simulink model "RLSim5"  (R2015b)
settings: Solver=ode45  StartTime=0.0  StopTime=16435  MaxStep=1  RelTol=1e-3
libraries: simulink x1
settings Model: Creator=jeff  LastModifiedBy=jeff
settings SolverCC: ZeroCrossAlgorithm=Adaptive
settings DataIOCC: SaveFormat=Array
settings DebuggingCC: IgnoredZcDiagnostic=none  SolverPrmCheckMsg=warning
settings HardwareCC: ProdBitPerPointer=32  ProdLargestAtomicFloat=None  ProdIntDivRoundTo=Undefined  ProdEndianess=Unspecified  ProdWordSize=32  ProdHWDeviceType=32-bit Generic
settings GRTTargetCC: GeneratePreprocessorConditionals=Disable all
settings ConfigComp: CovModelRefEnable=Off  CovSFcnEnable=off

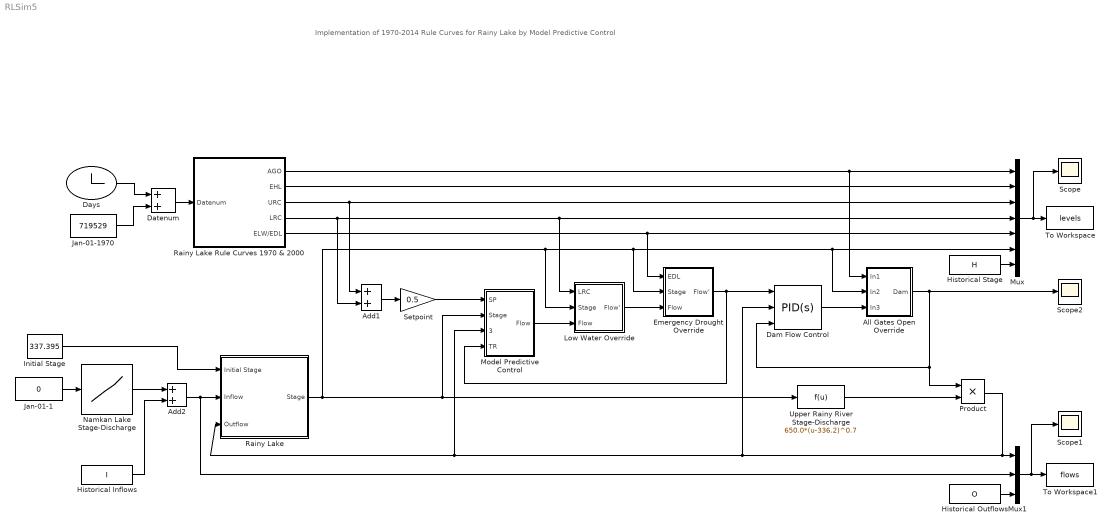
== system RLSim5 ==
  note: Implementation of 1970-2014 Rule Curves
      | for Rainy Lake by Model Predictive Control
  Add1 : Sum
  Add2 : Sum
  All Gates Open Override : Subsystem
  Dam Flow Control : simulink/Continuous/PID Controller (2DOF)  Controller=PID  TimeDomain=Continuous-time  SampleTime=-1  IntegratorMethod=Forward Euler  FilterMethod=Forward Euler  Form=Parallel  UseFilter=on  ControllerParametersSource=internal  P=0  I=0.00566146868750982  D=0  N=100  b=1  c=1  InitialConditionSource=internal  InitialConditionForIntegrator=0  InitialConditionForFilter=0  ExternalReset=none  LimitOutput=on  UpperSaturationLimit=1  LowerSaturationLimit=0  LinearizeAsGain=off  AntiWindupMode=clamping  Kb=1  TrackingMode=on  Kt=1  PParamMin=[]  PParamMax=[]  IParamMin=[]  IParamMax=[]  DParamMin=[]  DParamMax=[]  NParamMin=[]  NParamMax=[]  bParamMin=[]  bParamMax=[]  cParamMin=[]  cParamMax=[]  KbParamMin=[]  KbParamMax=[]  KtParamMin=[]  KtParamMax=[]  POutMin=[]  POutMax=[]  IOutMin=[]  IOutMax=[]  DOutMin=[]  DOutMax=[]  NOutMin=[]  NOutMax=[]  bOutMin=[]  bOutMax=[]  cOutMin=[]  cOutMax=[]  KbOutMin=[]  KbOutMax=[]  KtOutMin=[]  KtOutMax=[]  IntegratorOutMin=[]  IntegratorOutMax=[]  FilterOutMin=[]  FilterOutMax=[]  SumOutMin=[]  SumOutMax=[]  Sum1OutMin=[]  Sum1OutMax=[]  Sum2OutMin=[]  Sum2OutMax=[]  Sum3OutMin=[]  Sum3OutMax=[]  SumI1OutMin=[]  SumI1OutMax=[]  SumI2OutMin=[]  SumI2OutMax=[]  SumI3OutMin=[]  SumI3OutMax=[]  SumDOutMin=[]  SumDOutMax=[]  SaturationOutMin=[]  SaturationOutMax=[]  IntegratorContinuousStateAttributes=''  IntegratorStateMustResolveToSignalObject=off  IntegratorRTWStateStorageClass=Auto  FilterContinuousStateAttributes=''  FilterStateMustResolveToSignalObject=off  FilterRTWStateStorageClass=Auto  DifferentiatorICPrevScaledInput=0  DifferentiatorOutMin=[]  DifferentiatorOutMax=[]
  Datenum : Sum
  Days : Clock
  Emergency Drought Override : Subsystem
  Historical Inflows : FromWorkspace  VariableName=I  SampleTime=1
  Historical Outflows : FromWorkspace  VariableName=O  SampleTime=1
  Historical Stage : FromWorkspace  VariableName=H  SampleTime=1
  Initial Stage : Constant  Value=337.395
  Jan-01-1 : Constant  Value=0
  Jan-01-1970 : Constant  Value=719529
  Low Water Override : Subsystem
  Model Predictive Control : Subsystem
  Mux : Mux  Inputs=7
  Mux1 : Mux  Inputs=3
  Namkan Lake Stage-Discharge : Lookup_n-D  NumberOfTableDimensions=1  BreakpointsForDimension1=[335.21, 337.0, 338.0, 338.5, 339.0, 339.5, 340.0, 340.5, 341.0, 341.5, 342.0, 342.5, 343.0]  Table=[0 51 120 173 233 299 373 455 549 659 772 886 999]  ExtrapMethod=Clip  InternalRulePriority=Speed  RndMeth=Simplest  InputSameDT=on
  Product : Product
  Rainy Lake : Subsystem
  Rainy Lake Rule Curves 1970 & 2000 : Subsystem
  Scope : Scope
  Scope1 : Scope
  Scope2 : Scope
  Setpoint : Gain  Gain=0.5
  To Workspace : ToWorkspace  VariableName=levels  SaveFormat=Timeseries  SampleTime=-1
  To Workspace1 : ToWorkspace  VariableName=flows  SaveFormat=Timeseries  SampleTime=-1
  Upper Rainy River Stage-Discharge : Fcn  Expr=650.0*(u-336.2)^0.7
  wires:
  Days/1 -> Datenum/1
  Jan-01-1970/1 -> Datenum/2
  Datenum/1 -> Rainy Lake Rule Curves 1970 & 2000/1(Datenum)
  Mux/1 -> Scope/1, To Workspace/1
  Add1/1 -> Setpoint/1
  Rainy Lake Rule Curves 1970 & 2000/3(URC) -> Mux/3, Add1/1
  Initial Stage/1 -> Rainy Lake/1(Initial Stage)
  Mux1/1 -> Scope1/1, To Workspace1/1
  Rainy Lake Rule Curves 1970 & 2000/1(AGO) -> All Gates Open Override/1(In1), Mux/1
  Historical Stage/1 -> Mux/7
  Historical Outflows/1 -> Mux1/3
  Rainy Lake Rule Curves 1970 & 2000/2(EHL) -> Mux/2
  Add2/1 -> Mux1/2, Rainy Lake/2(Inflow)
  Namkan Lake Stage-Discharge/1 -> Add2/1
  Historical Inflows/1 -> Add2/2
  Jan-01-1/1 -> Namkan Lake Stage-Discharge/1
  Upper Rainy River Stage-Discharge/1 -> Product/2
  Product/1 -> Rainy Lake/3(Outflow), Model Predictive Control/3(Outflow), Dam Flow Control/2, Mux1/1
  Rainy Lake Rule Curves 1970 & 2000/5(ELW/EDL) -> Mux/5, Emergency Drought Override/1(EDL)
  Rainy Lake/1(Stage) -> Upper Rainy River Stage-Discharge/1, Model Predictive Control/2(Stage), Mux/6, All Gates Open Override/2(In2), Emergency Drought Override/2(Stage), Low Water Override/2(Stage)
  Low Water Override/1(Flow') -> Emergency Drought Override/3(Flow)
  Dam Flow Control/1 -> All Gates Open Override/3(In3)
  Emergency Drought Override/1(Flow') -> Dam Flow Control/1, Model Predictive Control/4(TR)
  Setpoint/1 -> Model Predictive Control/1(SP)
  Model Predictive Control/1(Flow) -> Low Water Override/3(Flow)
  Rainy Lake Rule Curves 1970 & 2000/4(LRC) -> Add1/2, Mux/4, Low Water Override/1(LRC)
  All Gates Open Override/1(Dam) -> Product/1, Dam Flow Control/3, Scope2/1

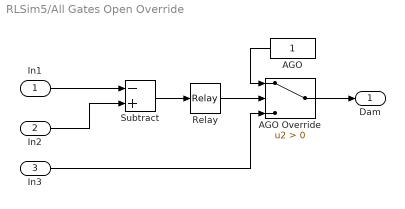
== system RLSim5/All Gates Open Override ==
  In1 : Inport
  In2 : Inport  Port=2
  In3 : Inport  Port=3
  AGO : Constant
  AGO Override : Switch  Criteria=u2 > Threshold
  Relay : Relay  OnSwitchValue=0.02  OffSwitchValue=-0.02
  Subtract : Sum  Inputs=-+
  Dam : Outport
  wires:
  Relay/1 -> AGO Override/2
  In3/1 -> AGO Override/3
  Subtract/1 -> Relay/1
  In2/1 -> Subtract/2
  AGO/1 -> AGO Override/1
  AGO Override/1 -> Dam/1
  In1/1 -> Subtract/1

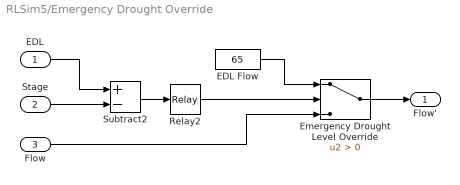
== system RLSim5/Emergency Drought Override ==
  EDL : Inport
  Stage : Inport  Port=2
  Flow : Inport  Port=3
  EDL Flow : Constant  Value=65
  Emergency Drought Level Override : Switch  Criteria=u2 > Threshold
  Relay2 : Relay  OnSwitchValue=0.02  OffSwitchValue=-0.02
  Subtract2 : Sum  Inputs=+-
  Flow' : Outport
  wires:
  Subtract2/1 -> Relay2/1
  Stage/1 -> Subtract2/2
  Emergency Drought Level Override/1 -> Flow'/1
  EDL Flow/1 -> Emergency Drought Level Override/1
  EDL/1 -> Subtract2/1
  Relay2/1 -> Emergency Drought Level Override/2
  Flow/1 -> Emergency Drought Level Override/3

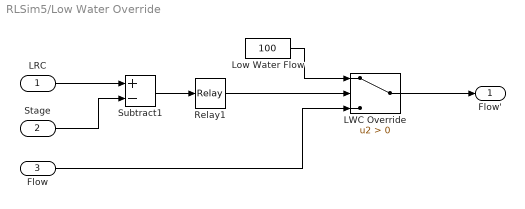
== system RLSim5/Low Water Override ==
  LRC : Inport
  Stage : Inport  Port=2
  Flow : Inport  Port=3
  LWC Override : Switch  Criteria=u2 > Threshold
  Low Water Flow : Constant  Value=100
  Relay1 : Relay  OnSwitchValue=0.02  OffSwitchValue=-0.02
  Subtract1 : Sum  Inputs=+-
  Flow' : Outport
  wires:
  Relay1/1 -> LWC Override/2
  Low Water Flow/1 -> LWC Override/1
  LWC Override/1 -> Flow'/1
  Subtract1/1 -> Relay1/1
  Flow/1 -> LWC Override/3
  LRC/1 -> Subtract1/1
  Stage/1 -> Subtract1/2

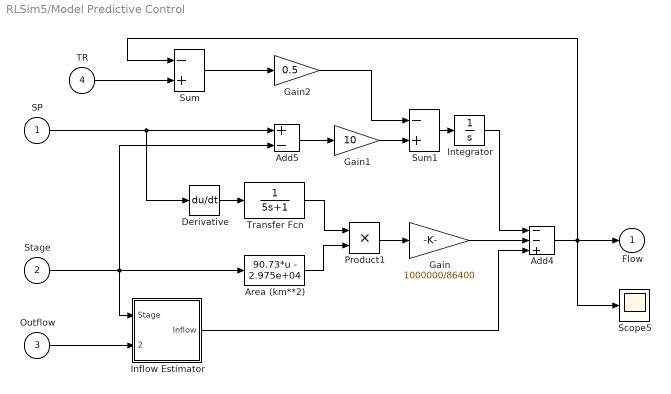
== system RLSim5/Model Predictive Control ==
  SP : Inport
  Stage : Inport  Port=2
  Outflow : Inport  Port=3
  TR : Inport  Port=4
  Add4 : Sum  Inputs=--+
  Add5 : Sum  Inputs=+-
  Area (km**2) : Fcn  Expr=90.73*u - 2.975e+04
  Derivative : Derivative  CoefficientInTFapproximation=Inf
  Gain : Gain  Gain=1000000/86400
  Gain1 : Gain  Gain=10
  Gain2 : Gain  Gain=0.5
  Inflow Estimator : Subsystem
  Integrator : Integrator
  Product1 : Product
  Scope5 : Scope
  Sum : Sum  Inputs=-+
  Sum1 : Sum  Inputs=-+
  Transfer Fcn : TransferFcn  Denominator=[5 1]
  Flow : Outport
  wires:
  Area (km**2)/1 -> Product1/2
  Stage/1 -> Add5/2, Area (km**2)/1, Inflow Estimator/1(Stage)
  SP/1 -> Derivative/1, Add5/1
  Add4/1 -> Flow/1, Scope5/1, Sum/1
  Add5/1 -> Gain1/1
  Product1/1 -> Gain/1
  Outflow/1 -> Inflow Estimator/2(Outflow)
  Derivative/1 -> Transfer Fcn/1
  Transfer Fcn/1 -> Product1/1
  Inflow Estimator/1(Inflow) -> Add4/3
  Gain/1 -> Add4/2
  Integrator/1 -> Add4/1
  TR/1 -> Sum/2
  Sum1/1 -> Integrator/1
  Gain1/1 -> Sum1/2
  Sum/1 -> Gain2/1
  Gain2/1 -> Sum1/1

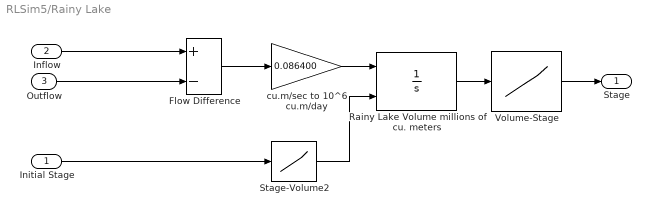
== system RLSim5/Rainy Lake ==
  Initial Stage : Inport
  Inflow : Inport  Port=2
  Outflow : Inport  Port=3
  Flow Difference : Sum  Inputs=+-
  Rainy Lake Volume millions of cu. meters : Integrator  InitialConditionSource=external  InitialCondition=1000  LimitOutput=on  LowerSaturationLimit=0  ContinuousStateAttributes='RainyLakeVolume'
  Stage-Volume2 : Lookup_n-D  NumberOfTableDimensions=1  BreakpointsForDimension1=[335.0 336.0 336.5 337.0 337.5 338.0 339.0 340.0]  Table=[112.67 798.00 1176.42 1577.25 2002.06 2450.57 3416.85 4458.97]  InternalRulePriority=Speed  RndMeth=Simplest  InputSameDT=on
  Volume-Stage : Lookup_n-D  NumberOfTableDimensions=1  BreakpointsForDimension1=[112.67 798.00 1176.42 1577.25 2002.06 2450.57 3416.85 4458.97]  Table=[335.0 336.0 336.5 337.0 337.5 338.0 339.0 340.0]  InternalRulePriority=Speed  RndMeth=Simplest  InputSameDT=on
  cu.m/sec to 10^6 cu.m/day : Gain  Gain=0.086400
  Stage : Outport
  wires:
  Outflow/1 -> Flow Difference/2
  Inflow/1 -> Flow Difference/1
  Rainy Lake Volume millions of cu. meters/1 -> Volume-Stage/1
  Stage-Volume2/1 -> Rainy Lake Volume millions of cu. meters/2
  cu.m/sec to 10^6 cu.m/day/1 -> Rainy Lake Volume millions of cu. meters/1
  Initial Stage/1 -> Stage-Volume2/1
  Volume-Stage/1 -> Stage/1
  Flow Difference/1 -> cu.m/sec to 10^6 cu.m/day/1

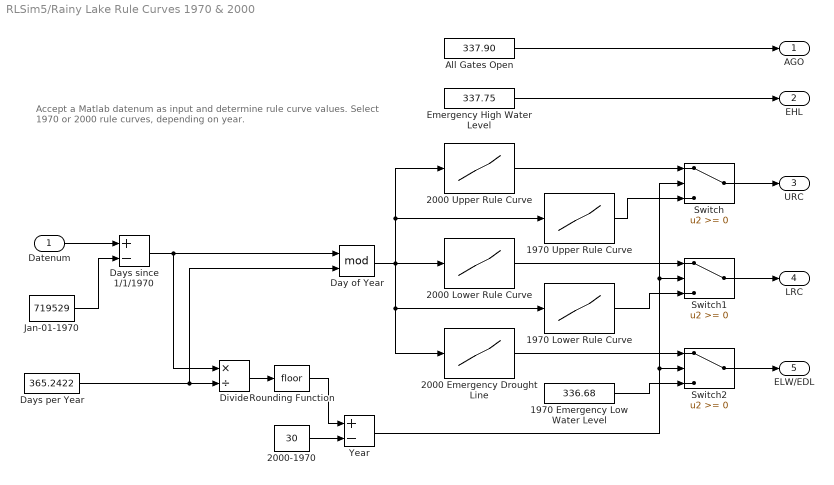
== system RLSim5/Rainy Lake Rule Curves 1970 & 2000 ==
  note: Accept a Matlab datenum as input and determine rule curve values. Select 1970 or 2000 rule curves, depending on year.
  Datenum : Inport
  1970 Emergency Low Water Level : Constant  Value=336.68
  1970 Lower Rule Curve : Lookup_n-D  NumberOfTableDimensions=1  BreakpointsForDimension1=[ 1 32 60 91 111 121 152 182 213 244 274 284 305 335 366]  Table=[ 337.30 337.05 336.87 336.69 336.69 336.84 337.30 337.54 337.54 337.54 337.54 337.54 337.48 337.36 337.23]  InternalRulePriority=Speed  RndMeth=Simplest  InputSameDT=on
  1970 Upper Rule Curve : Lookup_n-D  NumberOfTableDimensions=1  BreakpointsForDimension1=[ 1 32 60 91 111 121 152 182 213 244 274 284 305 335 365]  Table=[ 337.45 337.30 337.17 336.99 337.17 337.30 337.60 337.75 337.75 337.75 337.75 337.75 337.75 337.60 337.45]  InternalRulePriority=Speed  RndMeth=Simplest  InputSameDT=on
  2000 Emergency Drought Line : Lookup_n-D  NumberOfTableDimensions=1  BreakpointsForDimension1=[0 91 181 182 297 366]  Table=[336.90 336.70 336.70 337.20 337.20 336.90]  InternalRulePriority=Speed  RndMeth=Simplest  InputSameDT=on
  2000 Lower Rule Curve : Lookup_n-D  NumberOfTableDimensions=1  BreakpointsForDimension1=[0 91 121 152 182 227 335 366]  Table=[337.20 336.70 336.80 337.30 337.50 337.50 337.30 337.20]  InternalRulePriority=Speed  RndMeth=Simplest  InputSameDT=on
  2000 Upper Rule Curve : Lookup_n-D  NumberOfTableDimensions=1  BreakpointsForDimension1=[0 91 121 152 182 227 335 366]  Table="[337.45 337.0  337.40 337.60 337.75 337.75 337.60 337.45]"  InternalRulePriority=Speed  RndMeth=Simplest  InputSameDT=on
  2000-1970 : Constant  Value=30
  All Gates Open : Constant  Value=337.90
  Day of Year : Math  Operator=mod  SaturateOnIntegerOverflow=on
  Days per Year : Constant  Value=365.2422
  Days since 1/1/1970 : Sum  Inputs=+-
  Divide : Product  Inputs=*/
  Emergency High Water Level : Constant  Value=337.75
  Jan-01-1970 : Constant  Value=719529
  Rounding Function : Rounding
  Switch : Switch
  Switch1 : Switch
  Switch2 : Switch
  Year : Sum  Inputs=+-
  AGO : Outport
  EHL : Outport  Port=2
  URC : Outport  Port=3
  LRC : Outport  Port=4
  ELW/EDL : Outport  Port=5
  wires:
  Jan-01-1970/1 -> Days since 1/1/1970/2
  Days since 1/1/1970/1 -> Divide/1, Day of Year/1
  Days per Year/1 -> Day of Year/2, Divide/2
  Day of Year/1 -> 2000 Upper Rule Curve/1, 1970 Upper Rule Curve/1, 1970 Lower Rule Curve/1, 2000 Emergency Drought Line/1, 2000 Lower Rule Curve/1
  Datenum/1 -> Days since 1/1/1970/1
  All Gates Open/1 -> AGO/1
  2000 Emergency Drought Line/1 -> Switch2/1
  Emergency High Water Level/1 -> EHL/1
  Rounding Function/1 -> Year/1
  Divide/1 -> Rounding Function/1
  Switch/1 -> URC/1
  Switch1/1 -> LRC/1
  2000 Upper Rule Curve/1 -> Switch/1
  1970 Upper Rule Curve/1 -> Switch/3
  Switch2/1 -> ELW/EDL/1
  1970 Emergency Low Water Level/1 -> Switch2/3
  2000 Lower Rule Curve/1 -> Switch1/1
  1970 Lower Rule Curve/1 -> Switch1/3
  2000-1970/1 -> Year/2
  Year/1 -> Switch2/2, Switch1/2, Switch/2

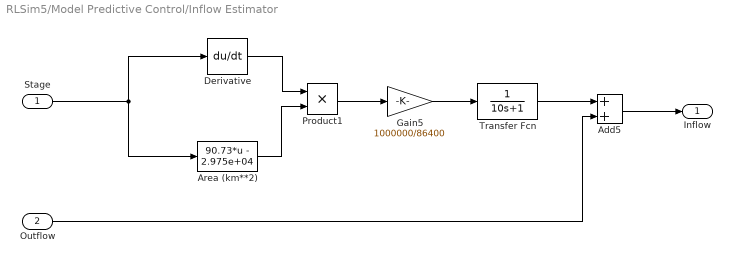
== system RLSim5/Model Predictive Control/Inflow Estimator ==
  Stage : Inport
  Outflow : Inport  Port=2
  Add5 : Sum
  Area (km**2) : Fcn  Expr=90.73*u - 2.975e+04
  Derivative : Derivative  CoefficientInTFapproximation=Inf
  Gain5 : Gain  Gain=1000000/86400
  Product1 : Product
  Transfer Fcn : TransferFcn  Denominator=[10 1]
  Inflow : Outport
  wires:
  Add5/1 -> Inflow/1
  Area (km**2)/1 -> Product1/2
  Stage/1 -> Area (km**2)/1, Derivative/1
  Derivative/1 -> Product1/1
  Product1/1 -> Gain5/1
  Gain5/1 -> Transfer Fcn/1
  Transfer Fcn/1 -> Add5/1
  Outflow/1 -> Add5/2
